simulink model "transformer_3"  (Simulink 7.4)
settings: Solver=ode23t  StartTime=0.0  StopTime=.2e-4  MaxStep=.5e-9  RelTol=1e-2
InitFcn:
  | L1=1e-6;
  | k  = 0.9;
  | N=2;
  | 
  | Lx=(1-k^2)*L1/(k^2)
  | 
  | M=N*L1;
  | L2=M^2/(L1*(k^2))
undefined symbols (not defined in the file or in its folder): Fs, gcbh, magnitude, powericon
libraries: powerlib x37, dspindex x24, dspsigops x12, dspbuff3 x8, dspxfrm3 x8, dsparch3 x8, dsparch4 x8, dspsnks4 x4, dspmtrx3 x4
(part 1 of 2)
settings Model: Creator=dbenson  LastModifiedBy=Dick
settings SolverCC: ZeroCrossControl=EnableAll
settings OptimizationCC: InitFltsAndDblsToZero=on
settings DebuggingCC: SaveWithParameterizedLinksMsg=none  SignalResolutionControl=TryResolveAllWithWarning  MultiTaskDSMMsg=warning  MultiTaskCondExecSysMsg=none
settings RTWCC: IncludeERTFirstTime=on
settings GRTTargetCC: TargetFcnLib=ansi_tfl_tmw.mat

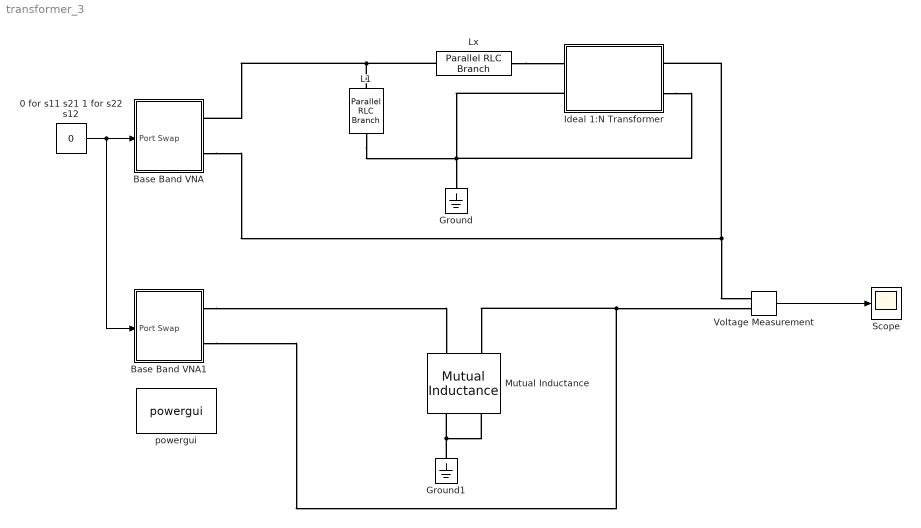
== system transformer_3 ==
  0 for s11 s21 1 for s22 s12 : Constant  Value=0  OutDataType=fixdt(1, 16)  OutScaling=2^0
  Base Band VNA : Subsystem  Description=Spectrum Analyzer  mask{BW=1e8, Frame_Size=256}
      mask prompts: BW "Bandwidth"; Frame_Size "FFT SIze (256,512,1024 etc)"
  Base Band VNA1 : Subsystem  Description=Spectrum Analyzer  mask{BW=1e8, Frame_Size=256}
      mask prompts: BW "Bandwidth"; Frame_Size "FFT SIze (256,512,1024 etc)"
  Ground : powerlib/Elements/Ground  DialogController=POWERSYS.PowerSysDialog  PhysicalDomain=powersysdomain  SubClassName=unknown  LeftPortType=p1  RightPortType=p1  LConnTagsString=a
  Ground1 : powerlib/Elements/Ground  DialogController=POWERSYS.PowerSysDialog  PhysicalDomain=powersysdomain  SubClassName=unknown  LeftPortType=p1  RightPortType=p1  LConnTagsString=a
  Ideal 1:N Transformer : Subsystem  mask{N=N}
      mask prompts: N "Turns Ratio Secondary/Primary"
  L1 : powerlib/Elements/Parallel RLC Branch  DialogController=POWERSYS.PowerSysDialog  PhysicalDomain=powersysdomain  SubClassName=unknown  LeftPortType=p1  RightPortType=p1  LConnTagsString=a  RConnTagsString=__new0  BranchType=L  Resistance=1  Inductance=L1  SetiL0=off  InitialCurrent=0  Capacitance=1e-6  Setx0=off  InitialVoltage=0  Measurements=None
  Lx : powerlib/Elements/Parallel RLC Branch  DialogController=POWERSYS.PowerSysDialog  PhysicalDomain=powersysdomain  SubClassName=unknown  LeftPortType=p1  RightPortType=p1  LConnTagsString=a  RConnTagsString=__new0  BranchType=RL  Resistance=1e6  Inductance=Lx  SetiL0=off  InitialCurrent=0  Capacitance=1e-6  Setx0=off  InitialVoltage=0  Measurements=None
  Mutual Inductance : powerlib/Elements/Mutual Inductance  DialogController=POWERSYS.PowerSysDialog  PhysicalDomain=powersysdomain  SubClassName=unknown  LeftPortType=p1  RightPortType=p1  LConnTagsString=a|b  RConnTagsString=A|B  TypeOfMutual=Two or three windings with equal mutual terms  NumberOfWindings=3  SelfImpedance1="[0.1    L1]"  SelfImpedance2="[0.1    L2]"  ThreeWindings=off  SelfImpedance3=[ 1.1 1.1e-03]  MutualImpedance="[0     M]"  InductanceMatrix="[1.0 0.9  0.9 ;  0.9 1.0  0.9;  0.9 0.9 1.0 ] * 1e-3"  ResistanceMatrix="[1.0 0.9  0.9 ;  0.9 1.0  0.9;  0.9 0.9 1.0 ]"  Measurements=None
      settings: AttributesFormatString=\n
  Scope : Scope
      settings: TimeRange=3e-006  YMin=-1.5  YMax=1.5
  Voltage Measurement : powerlib/Measurements/Voltage Measurement  DialogController=POWERSYS.PowerSysDialog  SystemSampleTime=-1  PhasorSimulation=off  OutputType=Complex  PSBequivalent=0
  powergui : powerlib/powergui  SystemSampleTime=-1  SimulationMode=Continuous  SampleTime=50e-6  frequency=60  SPID=off  DisableSnubberDevices=off  DisableRonSwitches=off  DisableVfSwitches=off  SwTol=0  Interpol=off  frequencyindice=0  echomessages=off  HookPort=off  DisplayEquations=off  FunctionMessages=off  EnableUseOfTLC=off  x0status=blocks  RestoreLinks=warning  Frange=[0:2:500]  Ylog=off  Xlog=on  ShowGrid=off  save=off  variable=ZData  ZoomFFT=on  StartTime=0.0  cycles=1  DisplayStyle=1  fundamental=60  FreqAxis=off  MaxFrequency=1000  frequencyindicesteady=1  RmsSteady=1  display=off  Ts=0  methode=off
  wires:
  0 for s11 s21 1 for s22 s12/1 -> Base Band VNA/1(Port Swap), Base Band VNA1/1(Port Swap)
  Voltage Measurement/1 -> Scope/1
  connections:
  Ideal 1:N Transformer/LConn2 -- Ground/LConn1 -- L1/RConn1 -- Ideal 1:N Transformer/RConn2
  L1/LConn1 -- Base Band VNA/RConn1 -- Lx/RConn1
  Base Band VNA/RConn2 -- Ideal 1:N Transformer/RConn1 -- Voltage Measurement/LConn1
  Lx/LConn1 -- Ideal 1:N Transformer/LConn1
  Base Band VNA1/RConn1 -- Mutual Inductance/LConn1
  Mutual Inductance/RConn2 -- Ground1/LConn1 -- Mutual Inductance/RConn1
  Base Band VNA1/RConn2 -- Mutual Inductance/LConn2 -- Voltage Measurement/LConn2

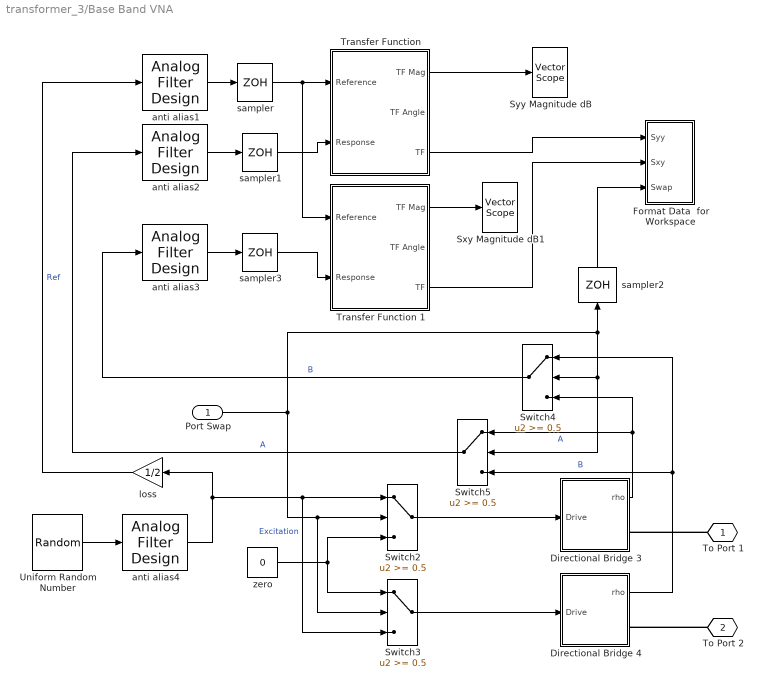
== system transformer_3/Base Band VNA ==
  Port Swap : Inport  OutDataType=sfix(16)  OutScaling=2^0
  Directional Bridge 3 : Subsystem  mask{Zo=50}
      mask prompts: Zo "Zo="
  Directional Bridge 4 : Subsystem  mask{Zo=50}
      mask prompts: Zo "Zo="
  Format Data  for Workspace : Subsystem
  Switch{2..5} (4 alike) : Switch  Threshold=0.5  SaturateOnIntegerOverflow=on
  Sxy Magnitude dB1 : dspsnks4/Vector Scope  DialogController=dspdialog.VectorScope  DialogControllerArgs=DataTag0  ScopeProperties=on  Domain=Frequency  HorizSpan=1  DisplayProperties=off  AxisGrid=on  Memory=off  FrameNumber=on  AxisLegend=off  AxisZoom=off  OpenScopeAtSimStart=on  OpenScopeImmediately=off  FigPos=[24 378 372 236]  AxisProperties=off  XUnits=Hertz  XRange=[0...Fs/2]  InheritXIncr=on  XIncr=2*Fs  XLabel=Time  XLimit=Auto  XMin=0  XMax=1  XStart=0  YUnits=dB  YLabel=dB  LineProperties=off  LineColors=[1 0 0]|[1 0 0]  XAxisParamsVer=6.9
      settings: YMin=-20  YMax=0
  Syy Magnitude dB : dspsnks4/Vector Scope  DialogController=dspdialog.VectorScope  DialogControllerArgs=DataTag1  ScopeProperties=on  Domain=Frequency  HorizSpan=1  DisplayProperties=off  AxisGrid=on  Memory=off  FrameNumber=on  AxisLegend=off  AxisZoom=off  OpenScopeAtSimStart=on  OpenScopeImmediately=off  FigPos=[24 92 372 236]  AxisProperties=off  XUnits=Hertz  XRange=[0...Fs/2]  InheritXIncr=on  XIncr=2*Fs  XLabel=Time  XLimit=Auto  XMin=0  XMax=1  XStart=0  YUnits=dB  YLabel=dB  LineProperties=off  LineColors=[1 0 0]|[1 0 0]  XAxisParamsVer=6.9
      settings: YMin=-20  YMax=0
  "Transfer Function " : Subsystem  mask{NFFT=Frame_Size, Navg=100, pcnt=100, unwrap_flag=on}
      mask prompts: NFFT "FFT length (power of 2):"; Navg "Spectral Averaging Factor (>=1):"; pcnt "Percentage of  Alias Free Data  (<=100)"; unwrap_flag "Unwrap Phase"
      mask Display: disp('Transfer Function \n Estimation (v2.0) ')
  Transfer Function 1 : Subsystem  mask{NFFT=Frame_Size, Navg=100, pcnt=100, unwrap_flag=on}
      mask prompts: NFFT "FFT length (power of 2):"; Navg "Spectral Averaging Factor (>=1):"; pcnt "Percentage of  Alias Free Data  (<=100)"; unwrap_flag "Unwrap Phase"
      mask Display: disp('Transfer Function \n Estimation (v2.0) ')
  Uniform Random Number : UniformRandomNumber  SampleTime=1/(2.56*BW)
  anti alias{1..4} (4 alike) : dsparch4/Analog Filter Design  method=Elliptic  filttype=Lowpass  N=8  Wlo=BW*2*pi  Whi=80  Rp=2  Rs=100
  loss : Gain  Gain=1/2  ParameterDataType=sfix(16)  ParameterScaling=2^0  OutDataType=sfix(16)  OutScaling=2^0  SaturateOnIntegerOverflow=on  OutDataTypeStr=Inherit: Same as input  ParamDataTypeStr=Inherit: Same as input
  sampler : ZeroOrderHold  SampleTime=1/(2.56*BW)
  sampler1 : ZeroOrderHold  SampleTime=1/(2.56*BW)
  sampler2 : ZeroOrderHold  SampleTime=256/(2.56*BW)
  sampler3 : ZeroOrderHold  SampleTime=1/(2.56*BW)
  zero : Constant  Value=0  OutDataType=sfix(16)  OutScaling=2^0
  To Port 1 : PMIOPort  Tag=PMCPort  Port=1  Side=Right
  To Port 2 : PMIOPort  Tag=PMCPort  Port=2  Side=Right
  wires:
  sampler/1 -> "Transfer Function "/1(Reference), Transfer Function 1/1(Reference)
  anti alias1/1 -> sampler/1
  anti alias2/1 -> sampler1/1
  Uniform Random Number/1 -> anti alias4/1
  anti alias3/1 -> sampler3/1
  sampler3/1 -> Transfer Function 1/2(Response)
  anti alias4/1 -> loss/1, Switch3/3, Switch2/1  "Excitation"
  loss/1 -> anti alias1/1  "Ref"
  Port Swap/1 -> Switch3/2, Switch2/2, Switch4/2, Switch5/2, sampler2/1
  zero/1 -> Switch2/3, Switch3/1
  Switch2/1 -> Directional Bridge 3/1(Drive)
  Switch3/1 -> Directional Bridge 4/1(Drive)
  Switch5/1 -> anti alias2/1  "A"
  Switch4/1 -> anti alias3/1  "B"
  Directional Bridge 3/1(rho) -> Switch4/3, Switch5/1  "A"
  Directional Bridge 4/1(rho) -> Switch5/3, Switch4/1  "B"
  sampler1/1 -> "Transfer Function "/2(Response)
  "Transfer Function "/1(TF Mag) -> Syy Magnitude dB/1
  Transfer Function 1/3("TF ") -> Format Data  for Workspace/2(Sxy)
  Transfer Function 1/1(TF Mag) -> Sxy Magnitude dB1/1
  "Transfer Function "/3("TF ") -> Format Data  for Workspace/1(Syy)
  sampler2/1 -> Format Data  for Workspace/3(Swap)
  connections:
  To Port 1/RConn1 -- Directional Bridge 3/RConn1
  To Port 2/RConn1 -- Directional Bridge 4/RConn1

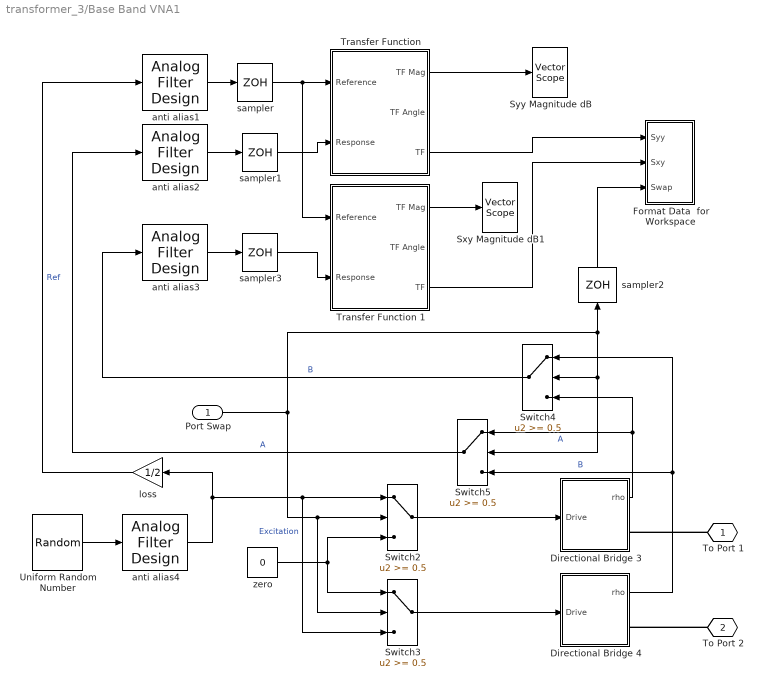
== system transformer_3/Base Band VNA1 ==
  Port Swap : Inport  OutDataType=sfix(16)  OutScaling=2^0
  Directional Bridge 3 : Subsystem  mask{Zo=50}
      mask prompts: Zo "Zo="
  Directional Bridge 4 : Subsystem  mask{Zo=50}
      mask prompts: Zo "Zo="
  Format Data  for Workspace : Subsystem
  Switch{2..5} (4 alike) : Switch  Threshold=0.5  SaturateOnIntegerOverflow=on
  Sxy Magnitude dB1 : dspsnks4/Vector Scope  DialogController=dspdialog.VectorScope  DialogControllerArgs=DataTag12  ScopeProperties=on  Domain=Frequency  HorizSpan=1  DisplayProperties=off  AxisGrid=on  Memory=off  FrameNumber=on  AxisLegend=off  AxisZoom=off  OpenScopeAtSimStart=on  OpenScopeImmediately=off  FigPos=[24 378 372 236]  AxisProperties=off  XUnits=Hertz  XRange=[0...Fs/2]  InheritXIncr=on  XIncr=2*Fs  XLabel=Time  XLimit=Auto  XMin=0  XMax=1  XStart=0  YUnits=dB  YLabel=dB  LineProperties=off  LineColors=[1 0 0]|[1 0 0]  XAxisParamsVer=6.9
      settings: YMin=-20  YMax=0
  Syy Magnitude dB : dspsnks4/Vector Scope  DialogController=dspdialog.VectorScope  DialogControllerArgs=DataTag13  ScopeProperties=on  Domain=Frequency  HorizSpan=1  DisplayProperties=off  AxisGrid=on  Memory=off  FrameNumber=on  AxisLegend=off  AxisZoom=off  OpenScopeAtSimStart=on  OpenScopeImmediately=off  FigPos=[24 92 372 236]  AxisProperties=off  XUnits=Hertz  XRange=[0...Fs/2]  InheritXIncr=on  XIncr=2*Fs  XLabel=Time  XLimit=Auto  XMin=0  XMax=1  XStart=0  YUnits=dB  YLabel=dB  LineProperties=off  LineColors=[1 0 0]|[1 0 0]  XAxisParamsVer=6.9
      settings: YMin=-20  YMax=0
  "Transfer Function " : Subsystem  mask{NFFT=Frame_Size, Navg=100, pcnt=100, unwrap_flag=on}
      mask prompts: NFFT "FFT length (power of 2):"; Navg "Spectral Averaging Factor (>=1):"; pcnt "Percentage of  Alias Free Data  (<=100)"; unwrap_flag "Unwrap Phase"
      mask Display: disp('Transfer Function \n Estimation (v2.0) ')
  Transfer Function 1 : Subsystem  mask{NFFT=Frame_Size, Navg=100, pcnt=100, unwrap_flag=on}
      mask prompts: NFFT "FFT length (power of 2):"; Navg "Spectral Averaging Factor (>=1):"; pcnt "Percentage of  Alias Free Data  (<=100)"; unwrap_flag "Unwrap Phase"
      mask Display: disp('Transfer Function \n Estimation (v2.0) ')
  Uniform Random Number : UniformRandomNumber  SampleTime=1/(2.56*BW)
  anti alias{1..4} (4 alike) : dsparch4/Analog Filter Design  method=Elliptic  filttype=Lowpass  N=8  Wlo=BW*2*pi  Whi=80  Rp=2  Rs=100
  loss : Gain  Gain=1/2  ParameterDataType=sfix(16)  ParameterScaling=2^0  OutDataType=sfix(16)  OutScaling=2^0  SaturateOnIntegerOverflow=on  OutDataTypeStr=Inherit: Same as input  ParamDataTypeStr=Inherit: Same as input
  sampler : ZeroOrderHold  SampleTime=1/(2.56*BW)
  sampler1 : ZeroOrderHold  SampleTime=1/(2.56*BW)
  sampler2 : ZeroOrderHold  SampleTime=256/(2.56*BW)
  sampler3 : ZeroOrderHold  SampleTime=1/(2.56*BW)
  zero : Constant  Value=0  OutDataType=sfix(16)  OutScaling=2^0
  To Port 1 : PMIOPort  Tag=PMCPort  Port=1  Side=Right
  To Port 2 : PMIOPort  Tag=PMCPort  Port=2  Side=Right
  wires:
  sampler2/1 -> Format Data  for Workspace/3(Swap)
  "Transfer Function "/3("TF ") -> Format Data  for Workspace/1(Syy)
  Transfer Function 1/1(TF Mag) -> Sxy Magnitude dB1/1
  Transfer Function 1/3("TF ") -> Format Data  for Workspace/2(Sxy)
  "Transfer Function "/1(TF Mag) -> Syy Magnitude dB/1
  sampler1/1 -> "Transfer Function "/2(Response)
  Directional Bridge 4/1(rho) -> Switch4/1, Switch5/3  "B"
  Directional Bridge 3/1(rho) -> Switch5/1, Switch4/3  "A"
  Switch4/1 -> anti alias3/1  "B"
  Switch5/1 -> anti alias2/1  "A"
  Switch3/1 -> Directional Bridge 4/1(Drive)
  Switch2/1 -> Directional Bridge 3/1(Drive)
  zero/1 -> Switch3/1, Switch2/3
  Port Swap/1 -> sampler2/1, Switch5/2, Switch4/2, Switch2/2, Switch3/2
  loss/1 -> anti alias1/1  "Ref"
  anti alias4/1 -> Switch2/1, Switch3/3, loss/1  "Excitation"
  sampler3/1 -> Transfer Function 1/2(Response)
  anti alias3/1 -> sampler3/1
  Uniform Random Number/1 -> anti alias4/1
  anti alias2/1 -> sampler1/1
  anti alias1/1 -> sampler/1
  sampler/1 -> Transfer Function 1/1(Reference), "Transfer Function "/1(Reference)
  connections:
  To Port 2/RConn1 -- Directional Bridge 4/RConn1
  To Port 1/RConn1 -- Directional Bridge 3/RConn1

== system transformer_3/Ideal 1:N Transformer ==
  CCS : powerlib/Electrical Sources/Controlled Current Source  Description=source block  DialogController=POWERSYS.PowerSysDialog  SystemSampleTime=-1  Initialize=off  Source_Type=AC  Amplitude=0  Phase=0  Frequency=0  Measurements=None
      settings: AttributesFormatString=\n
  CM : powerlib/Measurements/Current Measurement  Tag=PoWeRsYsTeMmEaSuReMeNt  DialogController=POWERSYS.PowerSysDialog  SystemSampleTime=-1  PhasorSimulation=off  OutputType=Magnitude  PSBequivalent=0
  CVS : powerlib/Electrical Sources/Controlled Voltage Source  Description=source block  DialogController=POWERSYS.PowerSysDialog  SystemSampleTime=-1  Initialize=off  Source_Type=AC  Amplitude=0  Phase=0  Frequency=0  Measurements=None
      settings: AttributesFormatString=\n
  Gain : Gain  Gain=-N  ParameterDataType=sfix(16)  ParameterScaling=2^0  OutDataType=sfix(16)  OutScaling=2^0  SaturateOnIntegerOverflow=on  OutDataTypeStr=Inherit: Same as input  ParamDataTypeStr=Inherit: Same as input
  Gain1 : Gain  Gain=N  ParameterDataType=sfix(16)  ParameterScaling=2^0  OutDataType=sfix(16)  OutScaling=2^0  SaturateOnIntegerOverflow=on  OutDataTypeStr=Inherit: Same as input  ParamDataTypeStr=Inherit: Same as input
  VM : powerlib/Measurements/Voltage Measurement  Tag=PoWeRsYsTeMmEaSuReMeNt  DialogController=POWERSYS.PowerSysDialog  SystemSampleTime=-1  PhasorSimulation=off  OutputType=Magnitude  PSBequivalent=0
  P1 : PMIOPort  Tag=PMCPort  Port=1  Side=Left
  P2 : PMIOPort  Tag=PMCPort  Port=2  Side=Left
  S1 : PMIOPort  Tag=PMCPort  Port=3  Side=Right
  S2 : PMIOPort  Tag=PMCPort  Port=4  Side=Right
  wires:
  CM/1 -> Gain/1
  Gain/1 -> CCS/1
  Gain1/1 -> CVS/1
  VM/1 -> Gain1/1
  connections:
  CVS/LConn1 -- S2/RConn1
  CM/RConn1 -- CVS/RConn1
  CM/LConn1 -- S1/RConn1
  CCS/RConn1 -- VM/LConn2 -- P2/RConn1
  CCS/LConn1 -- VM/LConn1 -- P1/RConn1

== system transformer_3/Base Band VNA/Directional Bridge 3 ==
  note: Directional Bridge
  Drive : Inport  OutDataType=sfix(16)  OutScaling=2^0
  CVS : powerlib/Electrical Sources/Controlled Voltage Source  Description=source block  DialogController=POWERSYS.PowerSysDialog  SystemSampleTime=-1  Initialize=off  Source_Type=AC  Amplitude=0  Phase=0  Frequency=0  Measurements=None
      settings: AttributesFormatString=\n
  G1 : powerlib/Elements/Ground  DialogController=POWERSYS.PowerSysDialog  PhysicalDomain=powersysdomain  SubClassName=unknown  LeftPortType=p1  RightPortType=p1  LConnTagsString=a
  G2 : powerlib/Elements/Ground  DialogController=POWERSYS.PowerSysDialog  PhysicalDomain=powersysdomain  SubClassName=unknown  LeftPortType=p1  RightPortType=p1  LConnTagsString=a
  R2 : powerlib/Elements/Series RLC Branch  DialogController=POWERSYS.PowerSysDialog  PhysicalDomain=powersysdomain  SubClassName=unknown  LeftPortType=p1  RightPortType=p1  LConnTagsString=__new0  RConnTagsString=__new0  BranchType=R  Resistance=Zo  Inductance=1.0  SetiL0=off  InitialCurrent=0  Capacitance=1.0  Setx0=off  InitialVoltage=0  Measurements=None
  R3 : powerlib/Elements/Series RLC Branch  DialogController=POWERSYS.PowerSysDialog  PhysicalDomain=powersysdomain  SubClassName=unknown  LeftPortType=p1  RightPortType=p1  LConnTagsString=__new0  RConnTagsString=__new0  BranchType=R  Resistance=Zo  Inductance=1.0  SetiL0=off  InitialCurrent=0  Capacitance=1.0  Setx0=off  InitialVoltage=0  Measurements=None
  R4 : powerlib/Elements/Series RLC Branch  DialogController=POWERSYS.PowerSysDialog  PhysicalDomain=powersysdomain  SubClassName=unknown  LeftPortType=p1  RightPortType=p1  LConnTagsString=__new0  RConnTagsString=__new0  BranchType=R  Resistance=Zo  Inductance=1.0  SetiL0=off  InitialCurrent=0  Capacitance=1.0  Setx0=off  InitialVoltage=0  Measurements=None
  VM : powerlib/Measurements/Voltage Measurement  Tag=PoWeRsYsTeMmEaSuReMeNt  DialogController=POWERSYS.PowerSysDialog  SystemSampleTime=-1  PhasorSimulation=off  OutputType=Magnitude  PSBequivalent=0
  Test Port : PMIOPort  Tag=PMCPort  Port=1  Side=Right
  rho : Outport  OutDataType=sfix(16)  OutScaling=2^0
  wires:
  VM/1 -> rho/1
  Drive/1 -> CVS/1
  connections:
  R2/RConn1 -- R3/LConn1 -- CVS/RConn1
  R4/LConn1 -- VM/LConn2 -- R2/LConn1
  G2/LConn1 -- R4/RConn1
  R3/RConn1 -- VM/LConn1 -- Test Port/RConn1
  G1/LConn1 -- CVS/LConn1

== system transformer_3/Base Band VNA/Directional Bridge 4 ==
  note: Directional Bridge
  Drive : Inport  OutDataType=sfix(16)  OutScaling=2^0
  CVS : powerlib/Electrical Sources/Controlled Voltage Source  Description=source block  DialogController=POWERSYS.PowerSysDialog  SystemSampleTime=-1  Initialize=off  Source_Type=AC  Amplitude=0  Phase=0  Frequency=0  Measurements=None
      settings: AttributesFormatString=\n
  G1 : powerlib/Elements/Ground  DialogController=POWERSYS.PowerSysDialog  PhysicalDomain=powersysdomain  SubClassName=unknown  LeftPortType=p1  RightPortType=p1  LConnTagsString=a
  G2 : powerlib/Elements/Ground  DialogController=POWERSYS.PowerSysDialog  PhysicalDomain=powersysdomain  SubClassName=unknown  LeftPortType=p1  RightPortType=p1  LConnTagsString=a
  R2 : powerlib/Elements/Series RLC Branch  DialogController=POWERSYS.PowerSysDialog  PhysicalDomain=powersysdomain  SubClassName=unknown  LeftPortType=p1  RightPortType=p1  LConnTagsString=__new0  RConnTagsString=__new0  BranchType=R  Resistance=Zo  Inductance=1.0  SetiL0=off  InitialCurrent=0  Capacitance=1.0  Setx0=off  InitialVoltage=0  Measurements=None
  R3 : powerlib/Elements/Series RLC Branch  DialogController=POWERSYS.PowerSysDialog  PhysicalDomain=powersysdomain  SubClassName=unknown  LeftPortType=p1  RightPortType=p1  LConnTagsString=__new0  RConnTagsString=__new0  BranchType=R  Resistance=Zo  Inductance=1.0  SetiL0=off  InitialCurrent=0  Capacitance=1.0  Setx0=off  InitialVoltage=0  Measurements=None
  R4 : powerlib/Elements/Series RLC Branch  DialogController=POWERSYS.PowerSysDialog  PhysicalDomain=powersysdomain  SubClassName=unknown  LeftPortType=p1  RightPortType=p1  LConnTagsString=__new0  RConnTagsString=__new0  BranchType=R  Resistance=Zo  Inductance=1.0  SetiL0=off  InitialCurrent=0  Capacitance=1.0  Setx0=off  InitialVoltage=0  Measurements=None
  VM : Subsystem  Tag=PoWeRsYsTeMmEaSuReMeNt  AncestorBlock=powerlib/Measurements/Voltage Measurement  LoadFcn=powericon('psbloadfunction',gcbh,'Measurement Block','');  InitFcn=powericon('psbloadfunction',gcbh,'InitFcnOfSPSBlocks','Measurement Block');  mask(Voltage Measurement){PhasorSimulation=off, OutputType=Magnitude, PSBequivalent=0}
      mask prompts: PhasorSimulation "Phasor simulation"; OutputType "Output signal :"; PSBequivalent "Equivalent circuit"
      mask help: Ideal voltage measurement.
      mask init:
      | switch OutputType
      | case 1
      |     OutputSelection = 1;
      |     NormalMode = 2;
      |     PhasorMode = 1;
      | case 2
      |     OutputSelection =[2,3];
      |     NormalMode = 3;
      |     PhasorMode = [1,2];
      | case 3
      |     OutputSelection =[4,5];
      |     NormalMode = 3;
      |     PhasorMode = [1,2];
      | case 4
      |     OutputSelection =[4];
      |     NormalMode = 2;
      |     PhasorMode = 1;
      | end
      | %
      | if PhasorSimulation
      |     SelectionMode = PhasorMode;
      | else
      |     SelectionMode = NormalMode;
      | end
      settings: AttributesFormatString=\n  CopyFcn=powericon('psbloadfunction',gcbh,'Measurement Block','VerifyPhasor');  PreSaveFcn=powericon('psbloadfunction',gcbh,'ModelCloseFcn','');  CloseFcn=powericon('psbloadfunction',gcbh,'CloseFcn','');
      mask Help: web(psbhelp);
      mask StyleString: checkbox,popup(Complex|Real-Imag|Magnitude-Angle|Magnitude),edit
  Test Port : PMIOPort  Tag=PMCPort  Port=1  Side=Right
  rho : Outport  OutDataType=sfix(16)  OutScaling=2^0
  wires:
  Drive/1 -> CVS/1
  VM/1(v) -> rho/1
  connections:
  G1/LConn1 -- CVS/LConn1
  Test Port/RConn1 -- VM/LConn1 -- R3/RConn1
  G2/LConn1 -- R4/RConn1
  R2/LConn1 -- VM/LConn2 -- R4/LConn1
  CVS/RConn1 -- R3/LConn1 -- R2/RConn1

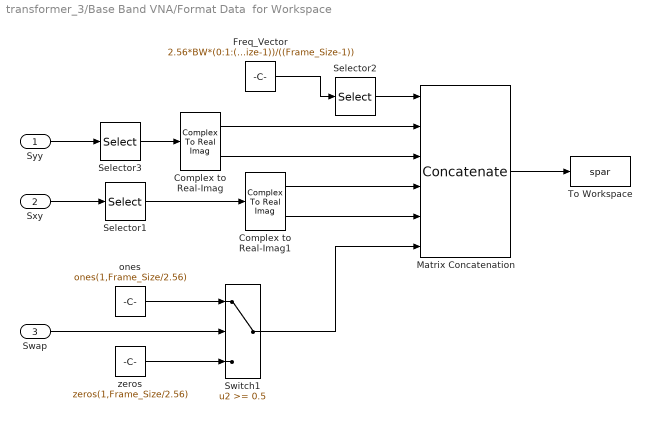
== system transformer_3/Base Band VNA/Format Data  for Workspace ==
  Syy : Inport  OutDataType=sfix(16)  OutScaling=2^0
  Sxy : Inport  Port=2  OutDataType=sfix(16)  OutScaling=2^0
  Swap : Inport  Port=3  OutDataType=sfix(16)  OutScaling=2^0
  Complex to Real-Imag : ComplexToRealImag
  Complex to Real-Imag1 : ComplexToRealImag
  Freq_Vector : Constant  Value=2.56*BW*(0:1:(Frame_Size-1))/((Frame_Size-1))  OutDataType=sfix(16)  OutScaling=2^0
  Matrix Concatenation : Concatenate  NumInputs=6  Mode=Multidimensional array  ConcatenateDimension=2
  Selector1 : Selector  InputPortWidth=Frame_Size  IndexOptions=Index vector (dialog)  Indices=[1:Frame_Size/2.56]  OutputSizes=1
  Selector2 : Selector  InputPortWidth=Frame_Size  IndexOptions=Index vector (dialog)  Indices=[1:Frame_Size/2.56]  OutputSizes=1
  Selector3 : Selector  InputPortWidth=Frame_Size  IndexOptions=Index vector (dialog)  Indices=[1:Frame_Size/2.56]  OutputSizes=1
  Switch1 : Switch  Threshold=0.5  SaturateOnIntegerOverflow=on
  To Workspace : ToWorkspace  VariableName=spar  SampleTime=-1  SaveFormat=Array
      settings: MaxDataPoints=1
  ones : Constant  Value=ones(1,Frame_Size/2.56)  OutDataType=sfix(16)  OutScaling=2^0
  zeros : Constant  Value=zeros(1,Frame_Size/2.56)  OutDataType=sfix(16)  OutScaling=2^0
  wires:
  Matrix Concatenation/1 -> To Workspace/1
  Complex to Real-Imag1/2 -> Matrix Concatenation/5
  Freq_Vector/1 -> Selector2/1
  Complex to Real-Imag/1 -> Matrix Concatenation/2
  Complex to Real-Imag/2 -> Matrix Concatenation/3
  Complex to Real-Imag1/1 -> Matrix Concatenation/4
  Syy/1 -> Selector3/1
  Sxy/1 -> Selector1/1
  ones/1 -> Switch1/1
  zeros/1 -> Switch1/3
  Swap/1 -> Switch1/2
  Switch1/1 -> Matrix Concatenation/6
  Selector3/1 -> Complex to Real-Imag/1
  Selector1/1 -> Complex to Real-Imag1/1
  Selector2/1 -> Matrix Concatenation/1

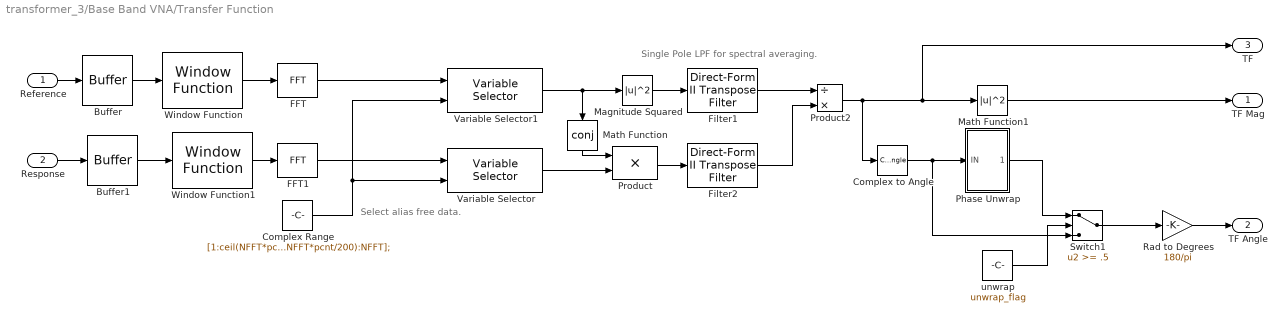
== system transformer_3/Base Band VNA/Transfer Function  ==
  note: Select alias free data.
  note: Single Pole LPF for spectral averaging.
  Reference : Inport  OutDataType=sfix(16)  OutScaling=2^0
  Response : Inport  Port=2  OutDataType=sfix(16)  OutScaling=2^0
  Buffer : dspbuff3/Buffer  N=NFFT  V=0  ic=0
  Buffer1 : dspbuff3/Buffer  N=NFFT  V=0  ic=0
  Complex Range : Constant  Value=[1:ceil(NFFT*pcnt/200),ceil(1+NFFT-NFFT*pcnt/200):NFFT];  OutDataType=sfix(16)  OutScaling=2^0
  Complex to Angle : ComplexToMagnitudeAngle  Output=Angle
  FFT : dspxfrm3/FFT  DialogController=dspDDGCreate  DialogControllerArgs=DataTag2  CompMethod=Table lookup  TableOpt=NEW  TableOptActive=Speed  BitRevOrder=off  InheritFFTLength=on  FFTLength=64  SkipNorm=on  firstCoeffMode=Specify word length  firstCoeffWordLength=16  firstCoeffFracLength=15  roundingMode=Floor  overflowMode=off
  FFT1 : dspxfrm3/FFT  DialogController=dspDDGCreate  DialogControllerArgs=DataTag3  CompMethod=Table lookup  TableOpt=NEW  TableOptActive=Speed  BitRevOrder=off  InheritFFTLength=on  FFTLength=64  SkipNorm=on  firstCoeffMode=User-defined  firstCoeffWordLength=16  firstCoeffFracLength=15  roundingMode=Floor  overflowMode=off
  Filter1 : dsparch3/Direct-Form II Transpose Filter  num=1  den=[Navg -(Navg-1)]  ic=eps
  Filter2 : dsparch3/Direct-Form II Transpose Filter  num=1  den=[Navg -(Navg-1)]  ic=eps
  Magnitude Squared : Math  Operator=magnitude^2  OutDataType=sfix(16)  OutScaling=2^0  SaturateOnIntegerOverflow=on
  Math Function : Math  Operator=conj  OutDataType=sfix(16)  OutScaling=2^0  SaturateOnIntegerOverflow=on
  Math Function1 : Math  Operator=magnitude^2  OutDataType=sfix(16)  OutScaling=2^0  SaturateOnIntegerOverflow=on
  Phase Unwrap : Subsystem
  Product : Product  OutDataType=sfix(16)  OutScaling=2^0  SaturateOnIntegerOverflow=on  InputSameDT=on  OutDataTypeStr=Inherit: Same as first input
  Product2 : Product  Inputs=/*  OutDataType=sfix(16)  OutScaling=2^0  SaturateOnIntegerOverflow=on  InputSameDT=on  OutDataTypeStr=Inherit: Same as first input
  Rad to Degrees : Gain  Gain=180/pi  ParameterDataType=sfix(16)  ParameterScaling=2^0  OutDataType=sfix(16)  OutScaling=2^0
  Switch1 : Switch  Threshold=.5
  Variable Selector : dspindex/Variable Selector  NumInputs=1  rowsOrCols=Rows  IdxMode=Variable  Elements=[1 3]  ZerOneIdxMode=One-based  errmode=Clip Index  FillMode=on  FillValues=0
  Variable Selector1 : dspindex/Variable Selector  NumInputs=1  rowsOrCols=Rows  IdxMode=Variable  Elements=[1 3]  ZerOneIdxMode=One-based  errmode=Clip Index  FillMode=on  FillValues=0
  Window Function : dspsigops/Window Function  DialogController=dspDDGCreate  DialogControllerArgs=DataTag5  winmode=Apply window to input  wintype=Hann  sampmode=Continuous  samptime=1  N=64  Rs=50  beta=10  winsamp=Periodic  UserWindow=hamming  OptParams=off  UserParams={'symmetric'}  dataType=double  isSigned=on  wordLen=16  udDataType=sfix(16)  fracBitsMode=Best precision  numFracBits=15  roundingMode=Floor  overflowMode=off  numSidelobes=4  sidelobeLevel=-30
  Window Function1 : dspsigops/Window Function  DialogController=dspDDGCreate  DialogControllerArgs=DataTag6  winmode=Apply window to input  wintype=Hann  sampmode=Continuous  samptime=1  N=64  Rs=50  beta=10  winsamp=Periodic  UserWindow=hamming  OptParams=off  UserParams={'symmetric'}  dataType=double  isSigned=on  wordLen=16  udDataType=sfix(16)  fracBitsMode=Best precision  numFracBits=15  roundingMode=Floor  overflowMode=off  numSidelobes=4  sidelobeLevel=-30
  unwrap : Constant  Value=unwrap_flag  OutDataType=sfix(16)  OutScaling=2^0
  TF Mag : Outport  OutDataType=sfix(16)  OutScaling=2^0
  TF Angle : Outport  Port=2  OutDataType=sfix(16)  OutScaling=2^0
  "TF " : Outport  Port=3  OutDataType=sfix(16)  OutScaling=2^0
  wires:
  Phase Unwrap/1(Out1) -> Switch1/1
  unwrap/1 -> Switch1/2
  Switch1/1 -> Rad to Degrees/1
  Variable Selector1/1 -> Math Function/1, Magnitude Squared/1
  Variable Selector/1 -> Product/2
  Product2/1 -> Complex to Angle/1, Math Function1/1, "TF "/1
  Buffer1/1 -> Window Function1/1
  Buffer/1 -> Window Function/1
  Filter2/1 -> Product2/2
  Filter1/1 -> Product2/1
  Window Function1/1 -> FFT1/1
  Window Function/1 -> FFT/1
  Math Function1/1 -> TF Mag/1
  FFT/1 -> Variable Selector1/1
  Magnitude Squared/1 -> Filter1/1
  Math Function/1 -> Product/1
  FFT1/1 -> Variable Selector/1
  Product/1 -> Filter2/1
  Reference/1 -> Buffer/1
  Response/1 -> Buffer1/1
  Rad to Degrees/1 -> TF Angle/1
  Complex to Angle/1 -> Phase Unwrap/1(IN), Switch1/3
  Complex Range/1 -> Variable Selector1/2, Variable Selector/2

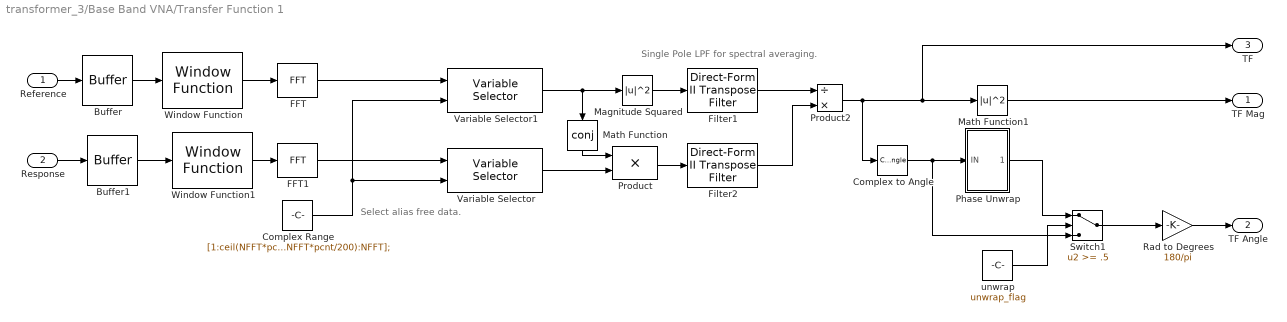
== system transformer_3/Base Band VNA/Transfer Function 1 ==
  note: Single Pole LPF for spectral averaging.
  note: Select alias free data.
  Reference : Inport  OutDataType=sfix(16)  OutScaling=2^0
  Response : Inport  Port=2  OutDataType=sfix(16)  OutScaling=2^0
  Buffer : dspbuff3/Buffer  N=NFFT  V=0  ic=0
  Buffer1 : dspbuff3/Buffer  N=NFFT  V=0  ic=0
  Complex Range : Constant  Value=[1:ceil(NFFT*pcnt/200),ceil(1+NFFT-NFFT*pcnt/200):NFFT];  OutDataType=sfix(16)  OutScaling=2^0
  Complex to Angle : ComplexToMagnitudeAngle  Output=Angle
  FFT : dspxfrm3/FFT  DialogController=dspDDGCreate  DialogControllerArgs=DataTag7  CompMethod=Table lookup  TableOpt=NEW  TableOptActive=Speed  BitRevOrder=off  InheritFFTLength=on  FFTLength=64  SkipNorm=on  firstCoeffMode=Specify word length  firstCoeffWordLength=16  firstCoeffFracLength=15  roundingMode=Floor  overflowMode=off
  FFT1 : dspxfrm3/FFT  DialogController=dspDDGCreate  DialogControllerArgs=DataTag8  CompMethod=Table lookup  TableOpt=NEW  TableOptActive=Speed  BitRevOrder=off  InheritFFTLength=on  FFTLength=64  SkipNorm=on  firstCoeffMode=User-defined  firstCoeffWordLength=16  firstCoeffFracLength=15  roundingMode=Floor  overflowMode=off
  Filter1 : dsparch3/Direct-Form II Transpose Filter  num=1  den=[Navg -(Navg-1)]  ic=eps
  Filter2 : dsparch3/Direct-Form II Transpose Filter  num=1  den=[Navg -(Navg-1)]  ic=eps
  Magnitude Squared : Math  Operator=magnitude^2  OutDataType=sfix(16)  OutScaling=2^0  SaturateOnIntegerOverflow=on
  Math Function : Math  Operator=conj  OutDataType=sfix(16)  OutScaling=2^0  SaturateOnIntegerOverflow=on
  Math Function1 : Math  Operator=magnitude^2  OutDataType=sfix(16)  OutScaling=2^0  SaturateOnIntegerOverflow=on
  Phase Unwrap : Subsystem
  Product : Product  OutDataType=sfix(16)  OutScaling=2^0  SaturateOnIntegerOverflow=on  InputSameDT=on  OutDataTypeStr=Inherit: Same as first input
  Product2 : Product  Inputs=/*  OutDataType=sfix(16)  OutScaling=2^0  SaturateOnIntegerOverflow=on  InputSameDT=on  OutDataTypeStr=Inherit: Same as first input
  Rad to Degrees : Gain  Gain=180/pi  ParameterDataType=sfix(16)  ParameterScaling=2^0  OutDataType=sfix(16)  OutScaling=2^0
  Switch1 : Switch  Threshold=.5
  Variable Selector : dspindex/Variable Selector  NumInputs=1  rowsOrCols=Rows  IdxMode=Variable  Elements=[1 3]  ZerOneIdxMode=One-based  errmode=Clip Index  FillMode=on  FillValues=0
  Variable Selector1 : dspindex/Variable Selector  NumInputs=1  rowsOrCols=Rows  IdxMode=Variable  Elements=[1 3]  ZerOneIdxMode=One-based  errmode=Clip Index  FillMode=on  FillValues=0
  Window Function : dspsigops/Window Function  DialogController=dspDDGCreate  DialogControllerArgs=DataTag10  winmode=Apply window to input  wintype=Hann  sampmode=Continuous  samptime=1  N=64  Rs=50  beta=10  winsamp=Periodic  UserWindow=hamming  OptParams=off  UserParams={'symmetric'}  dataType=double  isSigned=on  wordLen=16  udDataType=sfix(16)  fracBitsMode=Best precision  numFracBits=15  roundingMode=Floor  overflowMode=off  numSidelobes=4  sidelobeLevel=-30
  Window Function1 : dspsigops/Window Function  DialogController=dspDDGCreate  DialogControllerArgs=DataTag11  winmode=Apply window to input  wintype=Hann  sampmode=Continuous  samptime=1  N=64  Rs=50  beta=10  winsamp=Periodic  UserWindow=hamming  OptParams=off  UserParams={'symmetric'}  dataType=double  isSigned=on  wordLen=16  udDataType=sfix(16)  fracBitsMode=Best precision  numFracBits=15  roundingMode=Floor  overflowMode=off  numSidelobes=4  sidelobeLevel=-30
  unwrap : Constant  Value=unwrap_flag  OutDataType=sfix(16)  OutScaling=2^0
  TF Mag : Outport  OutDataType=sfix(16)  OutScaling=2^0
  TF Angle : Outport  Port=2  OutDataType=sfix(16)  OutScaling=2^0
  "TF " : Outport  Port=3  OutDataType=sfix(16)  OutScaling=2^0
  wires:
  Complex Range/1 -> Variable Selector/2, Variable Selector1/2
  Complex to Angle/1 -> Switch1/3, Phase Unwrap/1(IN)
  Rad to Degrees/1 -> TF Angle/1
  Response/1 -> Buffer1/1
  Reference/1 -> Buffer/1
  Product/1 -> Filter2/1
  FFT1/1 -> Variable Selector/1
  Math Function/1 -> Product/1
  Magnitude Squared/1 -> Filter1/1
  FFT/1 -> Variable Selector1/1
  Math Function1/1 -> TF Mag/1
  Window Function/1 -> FFT/1
  Window Function1/1 -> FFT1/1
  Filter1/1 -> Product2/1
  Filter2/1 -> Product2/2
  Buffer/1 -> Window Function/1
  Buffer1/1 -> Window Function1/1
  Product2/1 -> "TF "/1, Math Function1/1, Complex to Angle/1
  Variable Selector/1 -> Product/2
  Variable Selector1/1 -> Magnitude Squared/1, Math Function/1
  Switch1/1 -> Rad to Degrees/1
  unwrap/1 -> Switch1/2
  Phase Unwrap/1(Out1) -> Switch1/1

== system transformer_3/Base Band VNA1/Directional Bridge 3 ==
  note: Directional Bridge
  Drive : Inport  OutDataType=sfix(16)  OutScaling=2^0
  CVS : powerlib/Electrical Sources/Controlled Voltage Source  Description=source block  DialogController=POWERSYS.PowerSysDialog  SystemSampleTime=-1  Initialize=off  Source_Type=AC  Amplitude=0  Phase=0  Frequency=0  Measurements=None
      settings: AttributesFormatString=\n
  G1 : powerlib/Elements/Ground  DialogController=POWERSYS.PowerSysDialog  PhysicalDomain=powersysdomain  SubClassName=unknown  LeftPortType=p1  RightPortType=p1  LConnTagsString=a
  G2 : powerlib/Elements/Ground  DialogController=POWERSYS.PowerSysDialog  PhysicalDomain=powersysdomain  SubClassName=unknown  LeftPortType=p1  RightPortType=p1  LConnTagsString=a
  R2 : powerlib/Elements/Series RLC Branch  DialogController=POWERSYS.PowerSysDialog  PhysicalDomain=powersysdomain  SubClassName=unknown  LeftPortType=p1  RightPortType=p1  LConnTagsString=__new0  RConnTagsString=__new0  BranchType=R  Resistance=Zo  Inductance=1.0  SetiL0=off  InitialCurrent=0  Capacitance=1.0  Setx0=off  InitialVoltage=0  Measurements=None
  R3 : powerlib/Elements/Series RLC Branch  DialogController=POWERSYS.PowerSysDialog  PhysicalDomain=powersysdomain  SubClassName=unknown  LeftPortType=p1  RightPortType=p1  LConnTagsString=__new0  RConnTagsString=__new0  BranchType=R  Resistance=Zo  Inductance=1.0  SetiL0=off  InitialCurrent=0  Capacitance=1.0  Setx0=off  InitialVoltage=0  Measurements=None
  R4 : powerlib/Elements/Series RLC Branch  DialogController=POWERSYS.PowerSysDialog  PhysicalDomain=powersysdomain  SubClassName=unknown  LeftPortType=p1  RightPortType=p1  LConnTagsString=__new0  RConnTagsString=__new0  BranchType=R  Resistance=Zo  Inductance=1.0  SetiL0=off  InitialCurrent=0  Capacitance=1.0  Setx0=off  InitialVoltage=0  Measurements=None
  VM : powerlib/Measurements/Voltage Measurement  Tag=PoWeRsYsTeMmEaSuReMeNt  DialogController=POWERSYS.PowerSysDialog  SystemSampleTime=-1  PhasorSimulation=off  OutputType=Magnitude  PSBequivalent=0
  Test Port : PMIOPort  Tag=PMCPort  Port=1  Side=Right
  rho : Outport  OutDataType=sfix(16)  OutScaling=2^0
  wires:
  Drive/1 -> CVS/1
  VM/1 -> rho/1
  connections:
  G1/LConn1 -- CVS/LConn1
  Test Port/RConn1 -- VM/LConn1 -- R3/RConn1
  G2/LConn1 -- R4/RConn1
  R2/LConn1 -- VM/LConn2 -- R4/LConn1
  CVS/RConn1 -- R3/LConn1 -- R2/RConn1

== system transformer_3/Base Band VNA1/Directional Bridge 4 ==
  note: Directional Bridge
  Drive : Inport  OutDataType=sfix(16)  OutScaling=2^0
  CVS : powerlib/Electrical Sources/Controlled Voltage Source  Description=source block  DialogController=POWERSYS.PowerSysDialog  SystemSampleTime=-1  Initialize=off  Source_Type=AC  Amplitude=0  Phase=0  Frequency=0  Measurements=None
      settings: AttributesFormatString=\n
  G1 : powerlib/Elements/Ground  DialogController=POWERSYS.PowerSysDialog  PhysicalDomain=powersysdomain  SubClassName=unknown  LeftPortType=p1  RightPortType=p1  LConnTagsString=a
  G2 : powerlib/Elements/Ground  DialogController=POWERSYS.PowerSysDialog  PhysicalDomain=powersysdomain  SubClassName=unknown  LeftPortType=p1  RightPortType=p1  LConnTagsString=a
  R2 : powerlib/Elements/Series RLC Branch  DialogController=POWERSYS.PowerSysDialog  PhysicalDomain=powersysdomain  SubClassName=unknown  LeftPortType=p1  RightPortType=p1  LConnTagsString=__new0  RConnTagsString=__new0  BranchType=R  Resistance=Zo  Inductance=1.0  SetiL0=off  InitialCurrent=0  Capacitance=1.0  Setx0=off  InitialVoltage=0  Measurements=None
  R3 : powerlib/Elements/Series RLC Branch  DialogController=POWERSYS.PowerSysDialog  PhysicalDomain=powersysdomain  SubClassName=unknown  LeftPortType=p1  RightPortType=p1  LConnTagsString=__new0  RConnTagsString=__new0  BranchType=R  Resistance=Zo  Inductance=1.0  SetiL0=off  InitialCurrent=0  Capacitance=1.0  Setx0=off  InitialVoltage=0  Measurements=None
  R4 : powerlib/Elements/Series RLC Branch  DialogController=POWERSYS.PowerSysDialog  PhysicalDomain=powersysdomain  SubClassName=unknown  LeftPortType=p1  RightPortType=p1  LConnTagsString=__new0  RConnTagsString=__new0  BranchType=R  Resistance=Zo  Inductance=1.0  SetiL0=off  InitialCurrent=0  Capacitance=1.0  Setx0=off  InitialVoltage=0  Measurements=None
  VM : Subsystem  Tag=PoWeRsYsTeMmEaSuReMeNt  AncestorBlock=powerlib/Measurements/Voltage Measurement  LoadFcn=powericon('psbloadfunction',gcbh,'Measurement Block','');  InitFcn=powericon('psbloadfunction',gcbh,'InitFcnOfSPSBlocks','Measurement Block');  mask(Voltage Measurement){PhasorSimulation=off, OutputType=Magnitude, PSBequivalent=0}
      mask prompts: PhasorSimulation "Phasor simulation"; OutputType "Output signal :"; PSBequivalent "Equivalent circuit"
      mask help: Ideal voltage measurement.
      mask init: same as transformer_3/Base Band VNA/Directional Bridge 4/VM
      settings: AttributesFormatString=\n  CopyFcn=powericon('psbloadfunction',gcbh,'Measurement Block','VerifyPhasor');  PreSaveFcn=powericon('psbloadfunction',gcbh,'ModelCloseFcn','');  CloseFcn=powericon('psbloadfunction',gcbh,'CloseFcn','');
      mask Help: web(psbhelp);
      mask StyleString: checkbox,popup(Complex|Real-Imag|Magnitude-Angle|Magnitude),edit
  Test Port : PMIOPort  Tag=PMCPort  Port=1  Side=Right
  rho : Outport  OutDataType=sfix(16)  OutScaling=2^0
  wires:
  VM/1(v) -> rho/1
  Drive/1 -> CVS/1
  connections:
  R2/RConn1 -- R3/LConn1 -- CVS/RConn1
  R4/LConn1 -- VM/LConn2 -- R2/LConn1
  G2/LConn1 -- R4/RConn1
  R3/RConn1 -- VM/LConn1 -- Test Port/RConn1
  G1/LConn1 -- CVS/LConn1

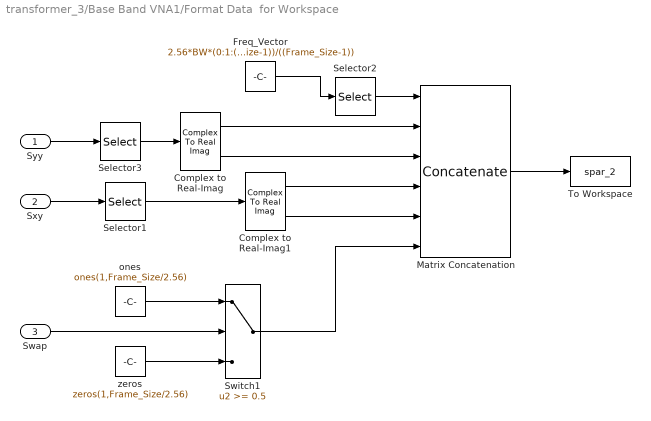
== system transformer_3/Base Band VNA1/Format Data  for Workspace ==
  Syy : Inport  OutDataType=sfix(16)  OutScaling=2^0
  Sxy : Inport  Port=2  OutDataType=sfix(16)  OutScaling=2^0
  Swap : Inport  Port=3  OutDataType=sfix(16)  OutScaling=2^0
  Complex to Real-Imag : ComplexToRealImag
  Complex to Real-Imag1 : ComplexToRealImag
  Freq_Vector : Constant  Value=2.56*BW*(0:1:(Frame_Size-1))/((Frame_Size-1))  OutDataType=sfix(16)  OutScaling=2^0
  Matrix Concatenation : Concatenate  NumInputs=6  Mode=Multidimensional array  ConcatenateDimension=2
  Selector1 : Selector  InputPortWidth=Frame_Size  IndexOptions=Index vector (dialog)  Indices=[1:Frame_Size/2.56]  OutputSizes=1
  Selector2 : Selector  InputPortWidth=Frame_Size  IndexOptions=Index vector (dialog)  Indices=[1:Frame_Size/2.56]  OutputSizes=1
  Selector3 : Selector  InputPortWidth=Frame_Size  IndexOptions=Index vector (dialog)  Indices=[1:Frame_Size/2.56]  OutputSizes=1
  Switch1 : Switch  Threshold=0.5  SaturateOnIntegerOverflow=on
  To Workspace : ToWorkspace  VariableName=spar_2  SampleTime=-1  SaveFormat=Array
      settings: MaxDataPoints=1
  ones : Constant  Value=ones(1,Frame_Size/2.56)  OutDataType=sfix(16)  OutScaling=2^0
  zeros : Constant  Value=zeros(1,Frame_Size/2.56)  OutDataType=sfix(16)  OutScaling=2^0
  wires:
  Selector2/1 -> Matrix Concatenation/1
  Selector1/1 -> Complex to Real-Imag1/1
  Selector3/1 -> Complex to Real-Imag/1
  Switch1/1 -> Matrix Concatenation/6
  Swap/1 -> Switch1/2
  zeros/1 -> Switch1/3
  ones/1 -> Switch1/1
  Sxy/1 -> Selector1/1
  Syy/1 -> Selector3/1
  Complex to Real-Imag1/1 -> Matrix Concatenation/4
  Complex to Real-Imag/2 -> Matrix Concatenation/3
  Complex to Real-Imag/1 -> Matrix Concatenation/2
  Freq_Vector/1 -> Selector2/1
  Complex to Real-Imag1/2 -> Matrix Concatenation/5
  Matrix Concatenation/1 -> To Workspace/1

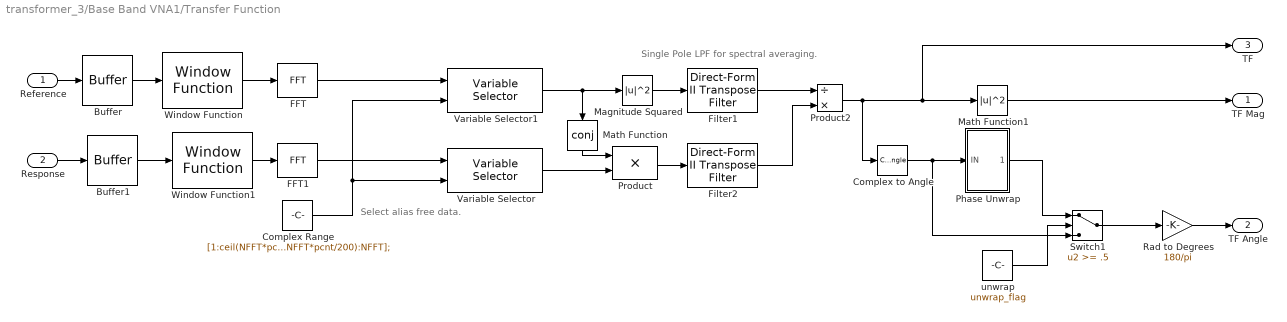
== system transformer_3/Base Band VNA1/Transfer Function  ==
  note: Single Pole LPF for spectral averaging.
  note: Select alias free data.
  Reference : Inport  OutDataType=sfix(16)  OutScaling=2^0
  Response : Inport  Port=2  OutDataType=sfix(16)  OutScaling=2^0
  Buffer : dspbuff3/Buffer  N=NFFT  V=0  ic=0
  Buffer1 : dspbuff3/Buffer  N=NFFT  V=0  ic=0
  Complex Range : Constant  Value=[1:ceil(NFFT*pcnt/200),ceil(1+NFFT-NFFT*pcnt/200):NFFT];  OutDataType=sfix(16)  OutScaling=2^0
  Complex to Angle : ComplexToMagnitudeAngle  Output=Angle
  FFT : dspxfrm3/FFT  DialogController=dspDDGCreate  DialogControllerArgs=DataTag14  CompMethod=Table lookup  TableOpt=NEW  TableOptActive=Speed  BitRevOrder=off  InheritFFTLength=on  FFTLength=64  SkipNorm=on  firstCoeffMode=Specify word length  firstCoeffWordLength=16  firstCoeffFracLength=15  roundingMode=Floor  overflowMode=off
  FFT1 : dspxfrm3/FFT  DialogController=dspDDGCreate  DialogControllerArgs=DataTag15  CompMethod=Table lookup  TableOpt=NEW  TableOptActive=Speed  BitRevOrder=off  InheritFFTLength=on  FFTLength=64  SkipNorm=on  firstCoeffMode=User-defined  firstCoeffWordLength=16  firstCoeffFracLength=15  roundingMode=Floor  overflowMode=off
  Filter1 : dsparch3/Direct-Form II Transpose Filter  num=1  den=[Navg -(Navg-1)]  ic=eps
  Filter2 : dsparch3/Direct-Form II Transpose Filter  num=1  den=[Navg -(Navg-1)]  ic=eps
  Magnitude Squared : Math  Operator=magnitude^2  OutDataType=sfix(16)  OutScaling=2^0  SaturateOnIntegerOverflow=on
  Math Function : Math  Operator=conj  OutDataType=sfix(16)  OutScaling=2^0  SaturateOnIntegerOverflow=on
  Math Function1 : Math  Operator=magnitude^2  OutDataType=sfix(16)  OutScaling=2^0  SaturateOnIntegerOverflow=on
  Phase Unwrap : Subsystem
  Product : Product  OutDataType=sfix(16)  OutScaling=2^0  SaturateOnIntegerOverflow=on  InputSameDT=on  OutDataTypeStr=Inherit: Same as first input
  Product2 : Product  Inputs=/*  OutDataType=sfix(16)  OutScaling=2^0  SaturateOnIntegerOverflow=on  InputSameDT=on  OutDataTypeStr=Inherit: Same as first input
  Rad to Degrees : Gain  Gain=180/pi  ParameterDataType=sfix(16)  ParameterScaling=2^0  OutDataType=sfix(16)  OutScaling=2^0
  Switch1 : Switch  Threshold=.5
  Variable Selector : dspindex/Variable Selector  NumInputs=1  rowsOrCols=Rows  IdxMode=Variable  Elements=[1 3]  ZerOneIdxMode=One-based  errmode=Clip Index  FillMode=on  FillValues=0
  Variable Selector1 : dspindex/Variable Selector  NumInputs=1  rowsOrCols=Rows  IdxMode=Variable  Elements=[1 3]  ZerOneIdxMode=One-based  errmode=Clip Index  FillMode=on  FillValues=0
  Window Function : dspsigops/Window Function  DialogController=dspDDGCreate  DialogControllerArgs=DataTag17  winmode=Apply window to input  wintype=Hann  sampmode=Continuous  samptime=1  N=64  Rs=50  beta=10  winsamp=Periodic  UserWindow=hamming  OptParams=off  UserParams={'symmetric'}  dataType=double  isSigned=on  wordLen=16  udDataType=sfix(16)  fracBitsMode=Best precision  numFracBits=15  roundingMode=Floor  overflowMode=off  numSidelobes=4  sidelobeLevel=-30
  Window Function1 : dspsigops/Window Function  DialogController=dspDDGCreate  DialogControllerArgs=DataTag18  winmode=Apply window to input  wintype=Hann  sampmode=Continuous  samptime=1  N=64  Rs=50  beta=10  winsamp=Periodic  UserWindow=hamming  OptParams=off  UserParams={'symmetric'}  dataType=double  isSigned=on  wordLen=16  udDataType=sfix(16)  fracBitsMode=Best precision  numFracBits=15  roundingMode=Floor  overflowMode=off  numSidelobes=4  sidelobeLevel=-30
  unwrap : Constant  Value=unwrap_flag  OutDataType=sfix(16)  OutScaling=2^0
  TF Mag : Outport  OutDataType=sfix(16)  OutScaling=2^0
  TF Angle : Outport  Port=2  OutDataType=sfix(16)  OutScaling=2^0
  "TF " : Outport  Port=3  OutDataType=sfix(16)  OutScaling=2^0
  wires:
  Complex Range/1 -> Variable Selector/2, Variable Selector1/2
  Complex to Angle/1 -> Switch1/3, Phase Unwrap/1(IN)
  Rad to Degrees/1 -> TF Angle/1
  Response/1 -> Buffer1/1
  Reference/1 -> Buffer/1
  Product/1 -> Filter2/1
  FFT1/1 -> Variable Selector/1
  Math Function/1 -> Product/1
  Magnitude Squared/1 -> Filter1/1
  FFT/1 -> Variable Selector1/1
  Math Function1/1 -> TF Mag/1
  Window Function/1 -> FFT/1
  Window Function1/1 -> FFT1/1
  Filter1/1 -> Product2/1
  Filter2/1 -> Product2/2
  Buffer/1 -> Window Function/1
  Buffer1/1 -> Window Function1/1
  Product2/1 -> "TF "/1, Math Function1/1, Complex to Angle/1
  Variable Selector/1 -> Product/2
  Variable Selector1/1 -> Magnitude Squared/1, Math Function/1
  Switch1/1 -> Rad to Degrees/1
  unwrap/1 -> Switch1/2
  Phase Unwrap/1(Out1) -> Switch1/1

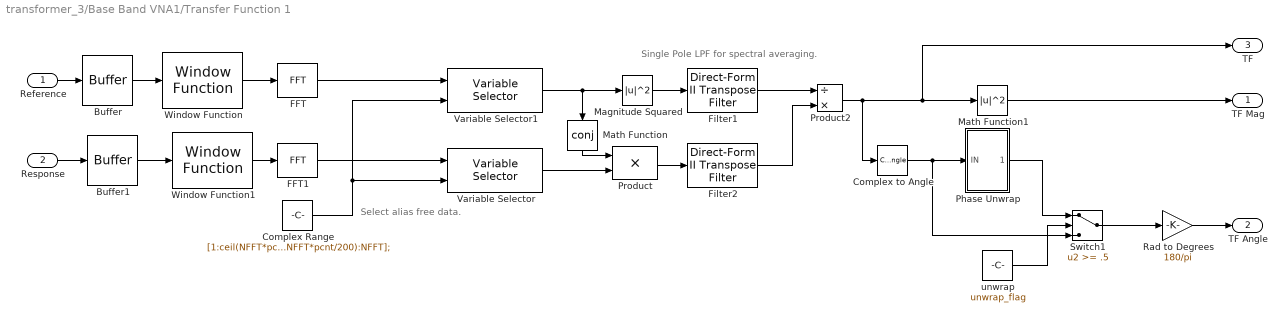
== system transformer_3/Base Band VNA1/Transfer Function 1 ==
  note: Select alias free data.
  note: Single Pole LPF for spectral averaging.
  Reference : Inport  OutDataType=sfix(16)  OutScaling=2^0
  Response : Inport  Port=2  OutDataType=sfix(16)  OutScaling=2^0
  Buffer : dspbuff3/Buffer  N=NFFT  V=0  ic=0
  Buffer1 : dspbuff3/Buffer  N=NFFT  V=0  ic=0
  Complex Range : Constant  Value=[1:ceil(NFFT*pcnt/200),ceil(1+NFFT-NFFT*pcnt/200):NFFT];  OutDataType=sfix(16)  OutScaling=2^0
  Complex to Angle : ComplexToMagnitudeAngle  Output=Angle
  FFT : dspxfrm3/FFT  DialogController=dspDDGCreate  DialogControllerArgs=DataTag19  CompMethod=Table lookup  TableOpt=NEW  TableOptActive=Speed  BitRevOrder=off  InheritFFTLength=on  FFTLength=64  SkipNorm=on  firstCoeffMode=Specify word length  firstCoeffWordLength=16  firstCoeffFracLength=15  roundingMode=Floor  overflowMode=off
  FFT1 : dspxfrm3/FFT  DialogController=dspDDGCreate  DialogControllerArgs=DataTag20  CompMethod=Table lookup  TableOpt=NEW  TableOptActive=Speed  BitRevOrder=off  InheritFFTLength=on  FFTLength=64  SkipNorm=on  firstCoeffMode=User-defined  firstCoeffWordLength=16  firstCoeffFracLength=15  roundingMode=Floor  overflowMode=off
  Filter1 : dsparch3/Direct-Form II Transpose Filter  num=1  den=[Navg -(Navg-1)]  ic=eps
  Filter2 : dsparch3/Direct-Form II Transpose Filter  num=1  den=[Navg -(Navg-1)]  ic=eps
  Magnitude Squared : Math  Operator=magnitude^2  OutDataType=sfix(16)  OutScaling=2^0  SaturateOnIntegerOverflow=on
  Math Function : Math  Operator=conj  OutDataType=sfix(16)  OutScaling=2^0  SaturateOnIntegerOverflow=on
  Math Function1 : Math  Operator=magnitude^2  OutDataType=sfix(16)  OutScaling=2^0  SaturateOnIntegerOverflow=on
  Phase Unwrap : Subsystem
  Product : Product  OutDataType=sfix(16)  OutScaling=2^0  SaturateOnIntegerOverflow=on  InputSameDT=on  OutDataTypeStr=Inherit: Same as first input
  Product2 : Product  Inputs=/*  OutDataType=sfix(16)  OutScaling=2^0  SaturateOnIntegerOverflow=on  InputSameDT=on  OutDataTypeStr=Inherit: Same as first input
  Rad to Degrees : Gain  Gain=180/pi  ParameterDataType=sfix(16)  ParameterScaling=2^0  OutDataType=sfix(16)  OutScaling=2^0
  Switch1 : Switch  Threshold=.5
  Variable Selector : dspindex/Variable Selector  NumInputs=1  rowsOrCols=Rows  IdxMode=Variable  Elements=[1 3]  ZerOneIdxMode=One-based  errmode=Clip Index  FillMode=on  FillValues=0
  Variable Selector1 : dspindex/Variable Selector  NumInputs=1  rowsOrCols=Rows  IdxMode=Variable  Elements=[1 3]  ZerOneIdxMode=One-based  errmode=Clip Index  FillMode=on  FillValues=0
  Window Function : dspsigops/Window Function  DialogController=dspDDGCreate  DialogControllerArgs=DataTag22  winmode=Apply window to input  wintype=Hann  sampmode=Continuous  samptime=1  N=64  Rs=50  beta=10  winsamp=Periodic  UserWindow=hamming  OptParams=off  UserParams={'symmetric'}  dataType=double  isSigned=on  wordLen=16  udDataType=sfix(16)  fracBitsMode=Best precision  numFracBits=15  roundingMode=Floor  overflowMode=off  numSidelobes=4  sidelobeLevel=-30
  Window Function1 : dspsigops/Window Function  DialogController=dspDDGCreate  DialogControllerArgs=DataTag23  winmode=Apply window to input  wintype=Hann  sampmode=Continuous  samptime=1  N=64  Rs=50  beta=10  winsamp=Periodic  UserWindow=hamming  OptParams=off  UserParams={'symmetric'}  dataType=double  isSigned=on  wordLen=16  udDataType=sfix(16)  fracBitsMode=Best precision  numFracBits=15  roundingMode=Floor  overflowMode=off  numSidelobes=4  sidelobeLevel=-30
  unwrap : Constant  Value=unwrap_flag  OutDataType=sfix(16)  OutScaling=2^0
  TF Mag : Outport  OutDataType=sfix(16)  OutScaling=2^0
  TF Angle : Outport  Port=2  OutDataType=sfix(16)  OutScaling=2^0
  "TF " : Outport  Port=3  OutDataType=sfix(16)  OutScaling=2^0
  wires:
  Phase Unwrap/1(Out1) -> Switch1/1
  unwrap/1 -> Switch1/2
  Switch1/1 -> Rad to Degrees/1
  Variable Selector1/1 -> Math Function/1, Magnitude Squared/1
  Variable Selector/1 -> Product/2
  Product2/1 -> Complex to Angle/1, Math Function1/1, "TF "/1
  Buffer1/1 -> Window Function1/1
  Buffer/1 -> Window Function/1
  Filter2/1 -> Product2/2
  Filter1/1 -> Product2/1
  Window Function1/1 -> FFT1/1
  Window Function/1 -> FFT/1
  Math Function1/1 -> TF Mag/1
  FFT/1 -> Variable Selector1/1
  Magnitude Squared/1 -> Filter1/1
  Math Function/1 -> Product/1
  FFT1/1 -> Variable Selector/1
  Product/1 -> Filter2/1
  Reference/1 -> Buffer/1
  Response/1 -> Buffer1/1
  Rad to Degrees/1 -> TF Angle/1
  Complex to Angle/1 -> Phase Unwrap/1(IN), Switch1/3
  Complex Range/1 -> Variable Selector1/2, Variable Selector/2

== system transformer_3/Base Band VNA/Directional Bridge 4/VM ==
  Mux : Mux  Inputs=2
  Phasor Measurements : Subsystem  TreatAsAtomicUnit=on
  Selector : Selector  InputPortWidth=length(OutputSelection)+1  IndexOptions=Index vector (dialog)  Indices=SelectionMode  OutputSizes=1
  Simulation method : Constant  Value=PhasorSimulation  OutDataType=sfix(16)  OutScaling=2^0
  VoltageMeasurement : PMComponent  PhysicalDomain=powersysdomain  LeftPortType=p1  RightPortType=p1  LConnTagsString=+  RConnTagsString=-
      mask Type: InnerPowersysBlock
  + : PMIOPort  Port=1  Side=Left
  - : PMIOPort  Port=2  Side=Left
  v : Outport  OutDataType=sfix(16)  OutScaling=2^0
  wires:
  Simulation method/1 -> Phasor Measurements/Enable
  Mux/1 -> Selector/1
  Phasor Measurements/1(options) -> Mux/1
  Selector/1 -> v/1
  [tpa9a03730_ff58_4815_ad5f_cd3660538f34] -> Phasor Measurements/1(measure), Mux/2
  connections:
  -/RConn1 -- VoltageMeasurement/RConn1
  +/RConn1 -- VoltageMeasurement/LConn1
